simulink model "DFIG_Wind_Vector_Control"  (R2024b)
settings: Solver=ode23t  StartTime=0.0  StopTime=50  RelTol=1e-3
undefined symbols (not defined in the file or in its folder): j
settings Model: Creator=Ioannis Vourkas  LastModifiedBy=Ioannis Vourkas

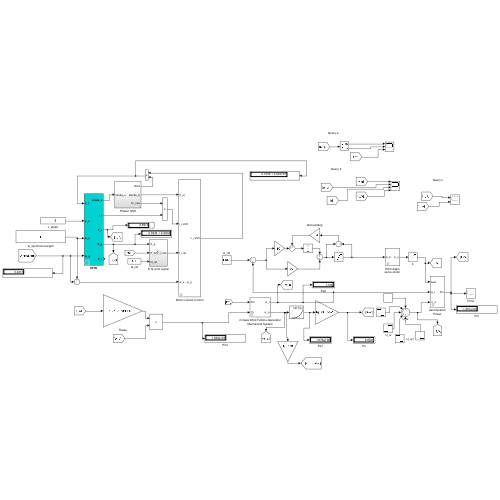
[thumbnail: Simulink's stored preview of the top-level diagram]
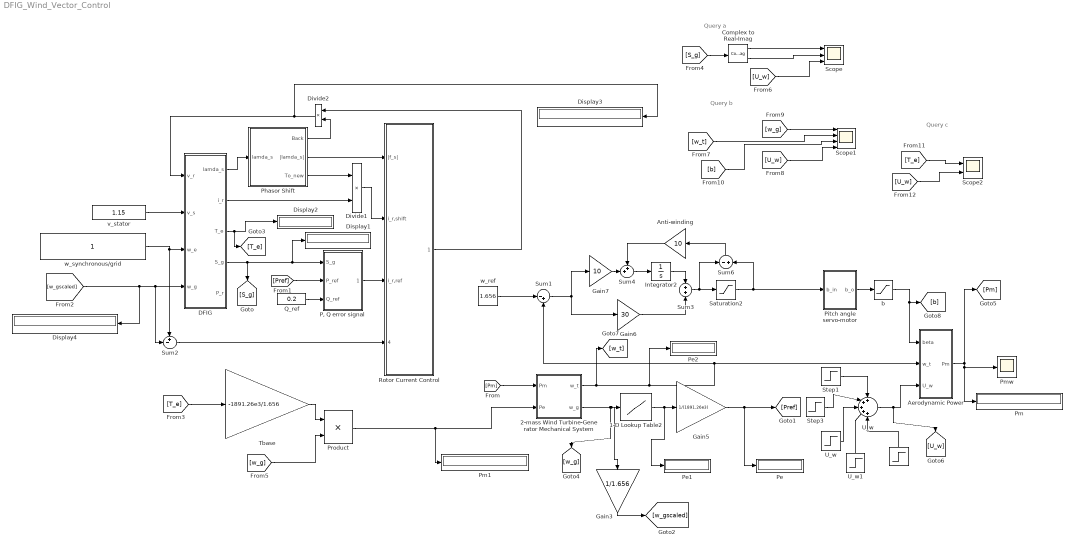
== system DFIG_Wind_Vector_Control ==
  note: Query a
  note: Query b
  note: Query c
  " " : Step  Time=35  After=-0.2  SampleTime=0
  " U_w" : Step  Time=20  After=0.45  SampleTime=0
  " U_w1" : Step  Time=25  After=-0.65  SampleTime=0
  1-D Lookup Table2 : Lookup_n-D  NumberOfTableDimensions=1  BreakpointsForDimension1=[0:0.05:1.656]  Table=416.257e3*[0:0.05:1.656].^3  InternalRulePriority=Speed  RndMeth=Simplest
  2-mass Wind Turbine-Generator Mechanical System : Subsystem  mask{K=15e6, D=5e6, Jt=8e6, Jn=100, w_init=1.656 %/(2*pi*60), w_inig=1.656 %/(2*pi*60)}
      mask prompts: K "Elasticity"; D "Damping"; Jt "Turb Moment of Inertia"; Jn "Gen Moment of Inertia"; w_init "Initial turb w"; w_inig "Initial gen w"
  Aerodynamic Power : Subsystem  mask{R=42, ro=1.225, z=[0.0045, 0.0290], c=[0.22, 116.00, 0.20, 0.00, 5.00, 12.20]}
      mask prompts: R "Radius"; ro "Air density"; z "Z parameters"; c "C parameters"
  Anti-winding : Gain  Gain=10
  Complex to Real-Imag : ComplexToRealImag
  DFIG : Subsystem  mask{R_s=(4.6+4/100)*0.001, R_r=3.8e-3, L_m=1.99, L_s=(118.18+4/20)*0.001}
  Display{1..4} (4 alike) : Display
  Divide1 : Product  Inputs=**
  Divide2 : Product  Inputs=**
  Gain3 : Gain  Gain=1/1.656
  Gain5 : Gain  Gain=1/(1891.26e3)
  Gain6 : Gain  Gain=30
  Gain7 : Gain  Gain=10
  Integrator2 : Integrator
  "P, Q error signal" : Subsystem
  Pe : Display
  Pe1 : Display
  Pe2 : Display
  Phasor Shift : Subsystem
  Pitch angle servo-motor : Subsystem  mask{Tpam=0.2}
      mask prompts: Tpam "Pitch angle motor"
  Pm : Display
  Pm1 : Display
  Pmw : Scope
  Product : Product
  Q_ref : Constant  Value=0.2
  Rotor Current Control : Subsystem  mask{R_r=3.8e-3, L_s=(118.18+4/20)*0.001, t_ir=1.1}
      mask prompts: t_ir "ir control time constant"
  Saturation2 : Saturate  UpperLimit=90  LowerLimit=0
  Scope : Scope  NumInputPorts=3
  Scope1 : Scope  NumInputPorts=4
  Scope2 : Scope  NumInputPorts=2
  Step1 : Step  Time=7  Before=10.7  After=11  SampleTime=0
  Step3 : Step  Time=13  Before=0.10  After=-0.5  SampleTime=0
  Sum1 : Sum  Inputs=|-+
  Sum2 : Sum  Inputs=+-|
  Sum3 : Sum  Inputs=+|+
  Sum4 : Sum  Inputs=++|
  Sum6 : Sum  Inputs=-|+
  Tbase : Gain  Gain=-1891.26e3/1.656
  U_w : Sum  Inputs=+++++
  b : Saturate  UpperLimit=90  LowerLimit=0
  v_stator : Constant  Value=1.15
  w_ref : Constant  Value=1.656
  w_synchronous/grid : Constant
  wires:
  DFIG/3(T_e) -> [T_e], Display2/1
  Phasor Shift/2(|lamda_s|) -> Rotor Current Control/1(|f_s|)
  "P, Q error signal"/1(i_r,ref) -> Rotor Current Control/3(i_r,ref)
  Q_ref/1 -> "P, Q error signal"/3(Q_ref)
  Sum2/1 -> Rotor Current Control/4(w_e - w_g)
  Divide2/1 -> DFIG/1(v_r), Display3/1
  Phasor Shift/1(Back) -> Divide2/2
  Rotor Current Control/1(v_r,shift) -> Divide2/1
  Divide1/1 -> Rotor Current Control/2(i_r,shift)
  DFIG/2(i_r) -> Divide1/2
  Phasor Shift/3(To_new) -> Divide1/1
  DFIG/1(lamda_s) -> Phasor Shift/1(lamda_s)
  [w_gscaled] -> DFIG/4(w_g), Sum2/2, Display4/1
  w_synchronous/grid/1 -> Sum2/1, DFIG/3(w_e)
  v_stator/1 -> DFIG/2(v_s)
  DFIG/4(S_g) -> [S_g], "P, Q error signal"/1(S_g), Display1/1
  U_w/1 -> [U_w], Aerodynamic Power/3(U_w)
  " "/1 -> U_w/5
  " U_w1"/1 -> U_w/4
  Step1/1 -> U_w/1
  " U_w"/1 -> U_w/3
  Step3/1 -> U_w/2
  1-D Lookup Table2/1 -> Pe1/1, Gain5/1
  [Pm] -> 2-mass Wind Turbine-Generator Mechanical System/1(Pm)
  Sum1/1 -> Gain7/1, Gain6/1
  Sum3/1 -> Sum6/1, Saturation2/1
  Pitch angle servo-motor/1(b_o) -> b/1
  Saturation2/1 -> Sum6/2, Pitch angle servo-motor/1(b_in)
  Sum4/1 -> Integrator2/1
  Anti-winding/1 -> Sum4/1
  b/1 -> [b], Aerodynamic Power/1(beta)
  Gain7/1 -> Sum4/2
  Integrator2/1 -> Sum3/1
  Gain6/1 -> Sum3/2
  Sum6/1 -> Anti-winding/1
  2-mass Wind Turbine-Generator Mechanical System/2(w_g) -> [w_g], Gain3/1, 1-D Lookup Table2/1
  [Pref] -> "P, Q error signal"/2(P_ref)
  w_ref/1 -> Sum1/1
  Gain3/1 -> [w_gscaled]
  [T_e] -> Tbase/1
  Gain5/1 -> Pe/1, [Pref]
  Product/1 -> Pm1/1, 2-mass Wind Turbine-Generator Mechanical System/2(Pe)
  Aerodynamic Power/1(Pm) -> Pm/1, Pmw/1, [Pm]
  2-mass Wind Turbine-Generator Mechanical System/1(w_t) -> [w_t], Pe2/1, Aerodynamic Power/2(w_t), Sum1/2
  Tbase/1 -> Product/1
  [w_g] -> Product/2
  [S_g] -> Complex to Real-Imag/1
  Complex to Real-Imag/1 -> Scope/1
  Complex to Real-Imag/2 -> Scope/2
  [U_w] -> Scope/3
  [U_w] -> Scope1/4
  [w_g] -> Scope1/1
  [w_t] -> Scope1/2
  [b] -> Scope1/3
  [U_w] -> Scope2/2
  [T_e] -> Scope2/1

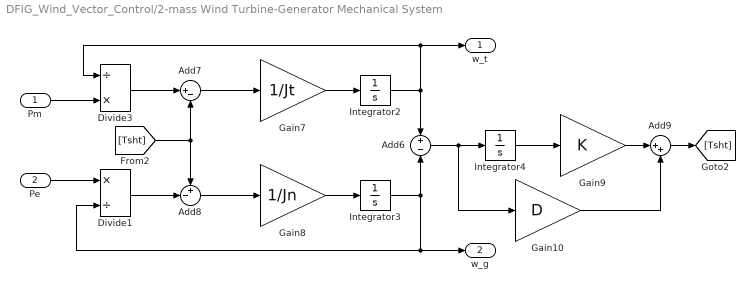
== system DFIG_Wind_Vector_Control/2-mass Wind Turbine-Generator Mechanical System ==
  Pm : Inport
  Pe : Inport  Port=2
  Add6 : Sum  Inputs=+|-
  Add7 : Sum  Inputs=|+-
  Add8 : Sum  Inputs=+-|
  Add9 : Sum  Inputs=|++
  Divide1 : Product  Inputs=*/
  Divide3 : Product  Inputs=/*
  Gain10 : Gain  Gain=D
  Gain7 : Gain  Gain=1/Jt
  Gain8 : Gain  Gain=1/Jn
  Gain9 : Gain  Gain=K
  Integrator2 : Integrator  InitialCondition=w_init
  Integrator3 : Integrator  InitialCondition=w_inig
  Integrator4 : Integrator  InitialCondition=0.35
  w_t : Outport
  w_g : Outport  Port=2
  wires:
  Add9/1 -> [Tsht]
  Gain8/1 -> Integrator3/1
  Integrator2/1 -> Add6/1, Divide3/1, w_t/1
  Gain7/1 -> Integrator2/1
  Add6/1 -> Gain10/1, Integrator4/1
  Integrator3/1 -> Divide1/2, w_g/1, Add6/2
  Integrator4/1 -> Gain9/1
  Divide1/1 -> Add8/2
  Gain10/1 -> Add9/2
  [Tsht] -> Add8/1, Add7/2
  Divide3/1 -> Add7/1
  Gain9/1 -> Add9/1
  Add8/1 -> Gain8/1
  Add7/1 -> Gain7/1
  Pe/1 -> Divide1/1
  Pm/1 -> Divide3/2

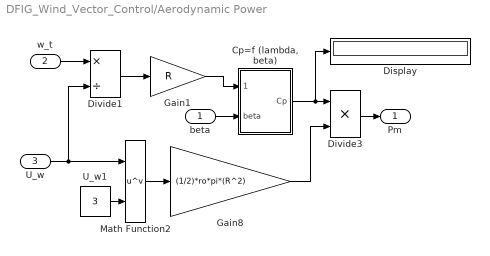
== system DFIG_Wind_Vector_Control/Aerodynamic Power ==
  beta : Inport
  w_t : Inport  Port=2
  U_w : Inport  Port=3
  "Cp=f (lambda, beta)" : Subsystem
  Display : Display
  Divide1 : Product  Inputs=*/
  Divide3 : Product  Inputs=**
  Gain1 : Gain  Gain=R
  Gain8 : Gain  Gain=(1/2)*ro*pi*(R^2)
  Math Function2 : Math  Operator=pow
  U_w1 : Constant  Value=3
  Pm : Outport
  wires:
  U_w/1 -> Divide1/2, Math Function2/1
  Math Function2/1 -> Gain8/1
  Divide3/1 -> Pm/1
  U_w1/1 -> Math Function2/2
  Gain8/1 -> Divide3/2
  "Cp=f (lambda, beta)"/1(Cp) -> Display/1, Divide3/1
  beta/1 -> "Cp=f (lambda, beta)"/2(beta)
  w_t/1 -> Divide1/1
  Divide1/1 -> Gain1/1
  Gain1/1 -> "Cp=f (lambda, beta)"/1(lambda)

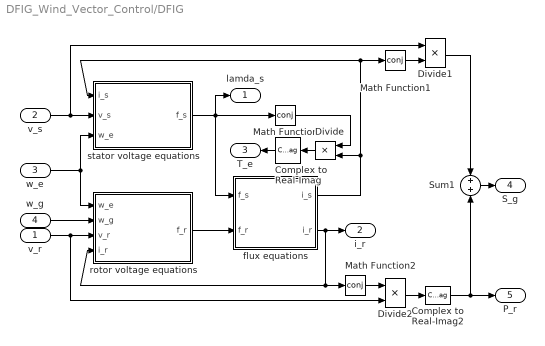
== system DFIG_Wind_Vector_Control/DFIG ==
  v_r : Inport
  v_s : Inport  Port=2
  w_e : Inport  Port=3
  w_g : Inport  Port=4
  Complex to Real-Imag : ComplexToRealImag  Output=Imag
  Complex to Real-Imag2 : ComplexToRealImag  Output=Real
  Divide : Product  Inputs=**
  Divide1 : Product  Inputs=**
  Divide2 : Product  Inputs=**
  Math Function : Math  Operator=conj  SignedPower=on
  Math Function1 : Math  Operator=conj  SignedPower=on
  Math Function2 : Math  Operator=conj  SignedPower=on
  Sum1 : Sum
  flux equations : Subsystem
  rotor voltage equations : Subsystem
  stator voltage equations : Subsystem
  lamda_s : Outport
  i_r : Outport  Port=2
  T_e : Outport  Port=3
  S_g : Outport  Port=4
  P_r : Outport  Port=5
  wires:
  Sum1/1 -> S_g/1
  w_g/1 -> rotor voltage equations/2(w_g)
  v_s/1 -> stator voltage equations/2(v_s), Divide1/1
  w_e/1 -> stator voltage equations/3(w_e), rotor voltage equations/1(w_e)
  v_r/1 -> Divide2/2, rotor voltage equations/3(v_r)
  flux equations/1(i_s) -> Math Function1/1, stator voltage equations/1(i_s), Divide/2
  flux equations/2(i_r) -> i_r/1, rotor voltage equations/4(i_r), Math Function2/1
  rotor voltage equations/1(f_r) -> flux equations/2(f_r)
  Divide/1 -> Complex to Real-Imag/1
  Complex to Real-Imag/1 -> T_e/1
  Math Function1/1 -> Divide1/2
  Divide1/1 -> Sum1/1
  Divide2/1 -> Complex to Real-Imag2/1
  Math Function/1 -> Divide/1
  stator voltage equations/1(f_s) -> Math Function/1, lamda_s/1, flux equations/1(f_s)
  Math Function2/1 -> Divide2/1
  Complex to Real-Imag2/1 -> Sum1/2, P_r/1

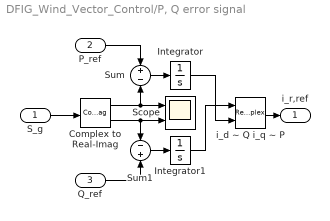
== system DFIG_Wind_Vector_Control/P, Q error signal ==
  S_g : Inport
  P_ref : Inport  Port=2
  Q_ref : Inport  Port=3
  Complex to Real-Imag : ComplexToRealImag
  Integrator : Integrator
  Integrator1 : Integrator
  Scope : Scope  NumInputPorts=2
  Sum : Sum  Inputs=+|-
  Sum1 : Sum  Inputs=-|+
  i_d ~ Q i_q ~ P : RealImagToComplex
  i_r,ref : Outport
  wires:
  S_g/1 -> Complex to Real-Imag/1
  P_ref/1 -> Sum/1
  Integrator1/1 -> i_d ~ Q i_q ~ P/1
  Sum1/1 -> Integrator1/1
  Q_ref/1 -> Sum1/2
  Integrator/1 -> i_d ~ Q i_q ~ P/2
  Complex to Real-Imag/1 -> Scope/1, Sum/2
  i_d ~ Q i_q ~ P/1 -> i_r,ref/1
  Complex to Real-Imag/2 -> Scope/2, Sum1/1
  Sum/1 -> Integrator/1

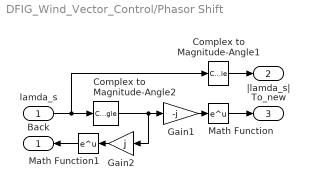
== system DFIG_Wind_Vector_Control/Phasor Shift ==
  lamda_s : Inport
  Complex to Magnitude-Angle1 : ComplexToMagnitudeAngle  Output=Magnitude
  Complex to Magnitude-Angle2 : ComplexToMagnitudeAngle  Output=Angle
  Gain1 : Gain  Gain=-j
  Gain2 : Gain  Gain=j
  Math Function : Math  SignedPower=on
  Math Function1 : Math  SignedPower=on
  Back : Outport
  |lamda_s| : Outport  Port=2
  To_new : Outport  Port=3
  wires:
  Complex to Magnitude-Angle1/1 -> |lamda_s|/1
  lamda_s/1 -> Complex to Magnitude-Angle2/1, Complex to Magnitude-Angle1/1
  Gain1/1 -> Math Function/1
  Gain2/1 -> Math Function1/1
  Math Function/1 -> To_new/1
  Math Function1/1 -> Back/1
  Complex to Magnitude-Angle2/1 -> Gain1/1, Gain2/1

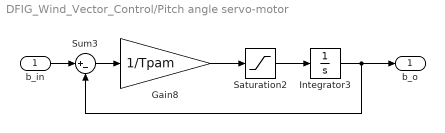
== system DFIG_Wind_Vector_Control/Pitch angle servo-motor ==
  b_in : Inport
  Gain8 : Gain  Gain=1/Tpam
  Integrator3 : Integrator
  Saturation2 : Saturate  UpperLimit=8  LowerLimit=-8
  Sum3 : Sum  Inputs=|+-
  b_o : Outport
  wires:
  Sum3/1 -> Gain8/1
  b_in/1 -> Sum3/1
  Gain8/1 -> Saturation2/1
  Integrator3/1 -> b_o/1, Sum3/2
  Saturation2/1 -> Integrator3/1

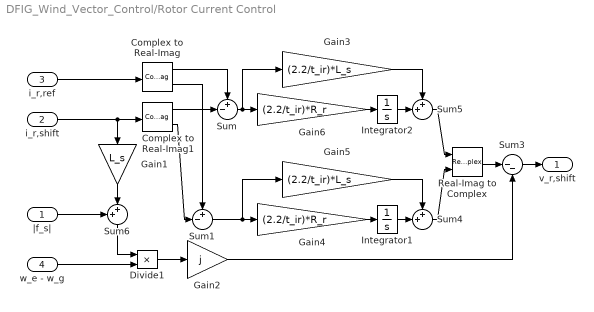
== system DFIG_Wind_Vector_Control/Rotor Current Control ==
  |f_s| : Inport
  i_r,shift : Inport  Port=2
  i_r,ref : Inport  Port=3
  w_e - w_g : Inport  Port=4
  Complex to Real-Imag : ComplexToRealImag
  Complex to Real-Imag1 : ComplexToRealImag
  Divide1 : Product  Inputs=**
  Gain1 : Gain  Gain=L_s
  Gain2 : Gain  Gain=j
  Gain3 : Gain  Gain=(2.2/t_ir)*L_s
  Gain4 : Gain  Gain=(2.2/t_ir)*R_r
  Gain5 : Gain  Gain=(2.2/t_ir)*L_s
  Gain6 : Gain  Gain=(2.2/t_ir)*R_r
  Integrator1 : Integrator
  Integrator2 : Integrator
  Real-Imag to Complex : RealImagToComplex
  Sum : Sum  Inputs=+-|
  Sum1 : Sum  Inputs=+-|
  Sum3 : Sum  Inputs=|--
  Sum4 : Sum  Inputs=++|
  Sum5 : Sum  Inputs=++|
  Sum6 : Sum  Inputs=++|
  v_r,shift : Outport
  wires:
  Sum/1 -> Gain6/1, Gain3/1
  i_r,ref/1 -> Complex to Real-Imag/1
  Complex to Real-Imag/1 -> Sum/1
  Complex to Real-Imag/2 -> Sum1/1
  i_r,shift/1 -> Complex to Real-Imag1/1, Gain1/1
  Complex to Real-Imag1/1 -> Sum/2
  Complex to Real-Imag1/2 -> Sum1/2
  w_e - w_g/1 -> Divide1/2
  Real-Imag to Complex/1 -> Sum3/1
  Sum3/1 -> v_r,shift/1
  Divide1/1 -> Gain2/1
  Integrator1/1 -> Sum4/2
  Gain4/1 -> Integrator1/1
  Sum1/1 -> Gain5/1, Gain4/1
  Integrator2/1 -> Sum5/2
  Gain6/1 -> Integrator2/1
  Sum5/1 -> Real-Imag to Complex/1
  Sum4/1 -> Real-Imag to Complex/2
  Gain5/1 -> Sum4/1
  Gain3/1 -> Sum5/1
  |f_s|/1 -> Sum6/1
  Gain1/1 -> Sum6/2
  Sum6/1 -> Divide1/1
  Gain2/1 -> Sum3/2

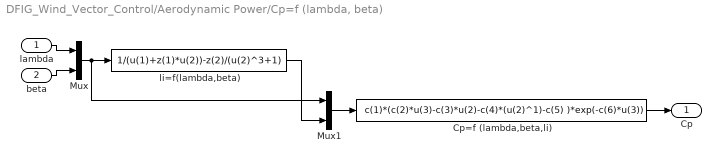
== system DFIG_Wind_Vector_Control/Aerodynamic Power/Cp=f (lambda, beta) ==
  lambda : Inport
  beta : Inport  Port=2
  Cp=f (lambda,beta,li) : Fcn  Expr=c(1)*(c(2)*u(3)-c(3)*u(2)-c(4)*(u(2)^1)-c(5) )*exp(-c(6)*u(3))  SampleTime=0
  Mux : Mux  Inputs=2
  Mux1 : Mux  Inputs=2
  li=f(lambda,beta) : Fcn  Expr=1/(u(1)+z(1)*u(2))-z(2)/(u(2)^3+1)  SampleTime=0
  Cp : Outport
  wires:
  Cp=f (lambda,beta,li)/1 -> Cp/1
  beta/1 -> Mux/2
  lambda/1 -> Mux/1
  li=f(lambda,beta)/1 -> Mux1/2
  Mux1/1 -> Cp=f (lambda,beta,li)/1
  Mux/1 -> Mux1/1, li=f(lambda,beta)/1

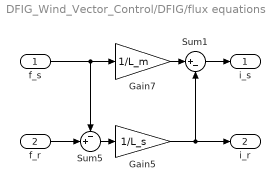
== system DFIG_Wind_Vector_Control/DFIG/flux equations ==
  f_s : Inport
  f_r : Inport  Port=2
  Gain5 : Gain  Gain=1/L_s
  Gain7 : Gain  Gain=1/L_m
  Sum1 : Sum  Inputs=|+-
  Sum5 : Sum  Inputs=-+|
  i_s : Outport
  i_r : Outport  Port=2
  wires:
  f_s/1 -> Gain7/1, Sum5/1
  Gain5/1 -> i_r/1, Sum1/2
  f_r/1 -> Sum5/2
  Sum5/1 -> Gain5/1
  Gain7/1 -> Sum1/1
  Sum1/1 -> i_s/1

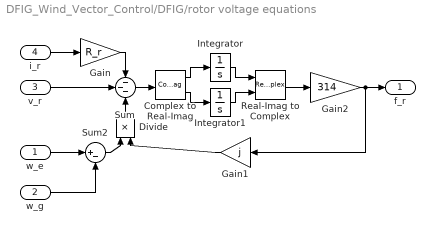
== system DFIG_Wind_Vector_Control/DFIG/rotor voltage equations ==
  w_e : Inport
  w_g : Inport  Port=2
  v_r : Inport  Port=3
  i_r : Inport  Port=4
  Complex to Real-Imag : ComplexToRealImag
  Divide : Product  Inputs=**
  Gain : Gain  Gain=R_r
  Gain1 : Gain  Gain=j
  Gain2 : Gain  Gain=314
  Integrator : Integrator
  Integrator1 : Integrator
  Real-Imag to Complex : RealImagToComplex
  Sum : Sum  Inputs=---
  Sum2 : Sum  Inputs=|+-
  f_r : Outport
  wires:
  Integrator/1 -> Real-Imag to Complex/1
  Integrator1/1 -> Real-Imag to Complex/2
  Divide/1 -> Sum/3
  Sum2/1 -> Divide/1
  Real-Imag to Complex/1 -> Gain2/1
  i_r/1 -> Gain/1
  v_r/1 -> Sum/2
  Gain/1 -> Sum/1
  w_e/1 -> Sum2/1
  w_g/1 -> Sum2/2
  Sum/1 -> Complex to Real-Imag/1
  Complex to Real-Imag/1 -> Integrator/1
  Complex to Real-Imag/2 -> Integrator1/1
  Gain1/1 -> Divide/2
  Gain2/1 -> f_r/1, Gain1/1

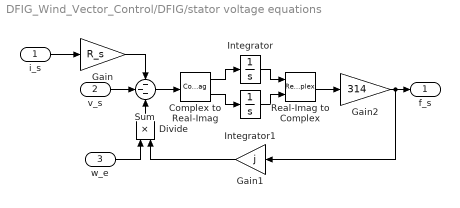
== system DFIG_Wind_Vector_Control/DFIG/stator voltage equations ==
  i_s : Inport
  v_s : Inport  Port=2
  w_e : Inport  Port=3
  Complex to Real-Imag : ComplexToRealImag
  Divide : Product  Inputs=**
  Gain : Gain  Gain=R_s
  Gain1 : Gain  Gain=j
  Gain2 : Gain  Gain=314
  Integrator : Integrator
  Integrator1 : Integrator
  Real-Imag to Complex : RealImagToComplex
  Sum : Sum  Inputs=---
  f_s : Outport
  wires:
  Integrator/1 -> Real-Imag to Complex/1
  Integrator1/1 -> Real-Imag to Complex/2
  Divide/1 -> Sum/3
  w_e/1 -> Divide/1
  Real-Imag to Complex/1 -> Gain2/1
  i_s/1 -> Gain/1
  Gain/1 -> Sum/1
  v_s/1 -> Sum/2
  Sum/1 -> Complex to Real-Imag/1
  Complex to Real-Imag/1 -> Integrator/1
  Complex to Real-Imag/2 -> Integrator1/1
  Gain1/1 -> Divide/2
  Gain2/1 -> f_s/1, Gain1/1
